simulink model "ABS_demo"  (R2022b)
settings: Solver=VariableStepAuto  StartTime=0.0  StopTime=25  RelTol=1e-3
undefined symbols (not defined in the file): g, I, m, R, v0
settings Model: Creator=Stephen Kingston  LastModifiedBy=OS
settings SolverCC: AlgebraicLoopSolver=TrustRegion
settings DebuggingCC: UnconnectedInputMsg=warning  UnconnectedOutputMsg=warning  UnconnectedLineMsg=warning  SFMachineParentedDataDiag=warning
settings ModelReferenceCC: EnableRefExpFcnMdlSchedulingChecks=on
settings SFSimCC: CustomCodeUndefinedFunction=UseInterfaceOnly

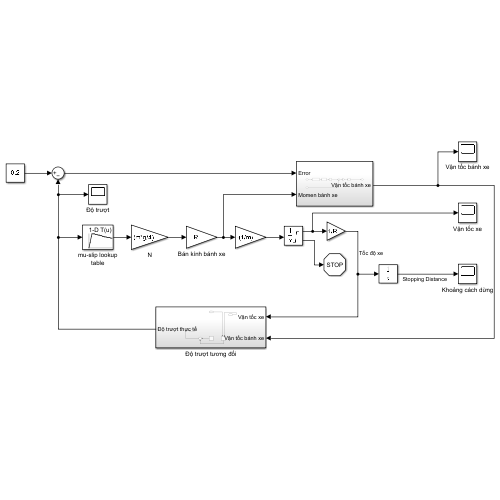
[thumbnail: Simulink's stored preview of the top-level diagram]
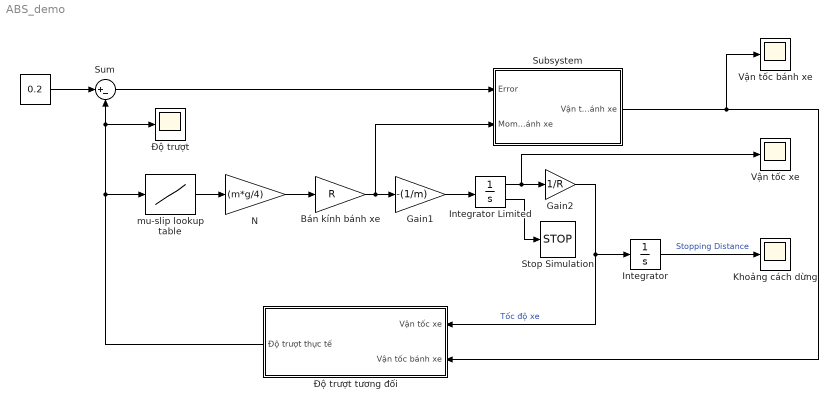
== system ABS_demo ==
  " " : Constant  Value=0.2
  Bán kính bánh xe : Gain  Gain=R
  Gain1 : Gain  Gain=-(1/m)
  Gain2 : Gain  Gain=1/R
  Integrator : Integrator
  Integrator Limited : Integrator  InitialCondition=v0  LimitOutput=on  UpperSaturationLimit=1000  LowerSaturationLimit=0  ShowSaturationPort=on
  Khoảng cách dừng : Scope
  N : Gain  Gain=(m*g/4)
  Stop Simulation : Stop
  Subsystem : Subsystem
  Sum : Sum  Inputs=|+-
  Vận tốc bánh xe : Scope
  Vận tốc xe : Scope
  mu-slip lookup table : Lookup_n-D  NumberOfTableDimensions=1  BreakpointsForDimension1=[0,0.05,0.1,0.15,0.2,0.25,0.3,0.35,0.4,0.45,0.5,0.55,0.60,0.65,0.70,0.75,0.80,0.85,0.90,0.95,1]  Table=[0,0.4,0.8,0.97,1,0.98,0.96,0.94,0.92,0.9,0.88,0.855,0.83,0.81,0.79,0.77,0.75,0.73,0.72,0.71,0.7]  InternalRulePriority=Speed  RndMeth=Simplest
  "Độ trượt " : Scope
  Độ trượt tương đối : Subsystem
  wires:
  Sum/1 -> Subsystem/1(Error)
  Bán kính bánh xe/1 -> Gain1/1, Subsystem/2(Momen bánh xe)
  Gain2/1 -> Độ trượt tương đối/1(Vận tốc xe), Integrator/1  "Tốc độ xe"
  " "/1 -> Sum/1
  mu-slip lookup table/1 -> N/1
  N/1 -> Bán kính bánh xe/1
  Gain1/1 -> Integrator Limited/1
  Integrator Limited/1 -> Vận tốc xe/1, Gain2/1
  Integrator/1 -> Khoảng cách dừng/1  "Stopping Distance"
  Integrator Limited/2 -> Stop Simulation/1
  Subsystem/1(Vận tốc bánh xe) -> Vận tốc bánh xe/1, Độ trượt tương đối/2(Vận tốc bánh xe)
  Độ trượt tương đối/1(Độ trượt thực tế) -> "Độ trượt "/1, Sum/2, mu-slip lookup table/1

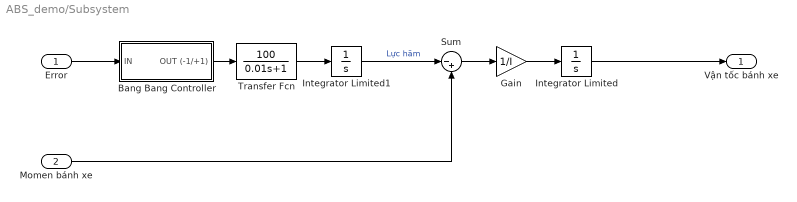
== system ABS_demo/Subsystem ==
  Error : Inport
  Momen bánh xe : Inport  Port=2
  Bang Bang Controller : Subsystem
  Gain : Gain  Gain=1/I
  Integrator Limited : Integrator  InitialCondition=v0/R  LimitOutput=on  UpperSaturationLimit=1000  LowerSaturationLimit=0
  Integrator Limited1 : Integrator  LimitOutput=on  UpperSaturationLimit=1500  LowerSaturationLimit=0
  Sum : Sum  Inputs=|-+
  Transfer Fcn : TransferFcn  Numerator=[100]  Denominator=[0.01 1]
  Vận tốc bánh xe : Outport  VectorParamsAs1DForOutWhenUnconnected=off
  wires:
  Sum/1 -> Gain/1
  Transfer Fcn/1 -> Integrator Limited1/1
  Gain/1 -> Integrator Limited/1
  Integrator Limited/1 -> Vận tốc bánh xe/1
  Integrator Limited1/1 -> Sum/1  "Lực hãm"
  Bang Bang Controller/1(OUT (-1/+1)) -> Transfer Fcn/1
  Momen bánh xe/1 -> Sum/2
  Error/1 -> Bang Bang Controller/1(IN)

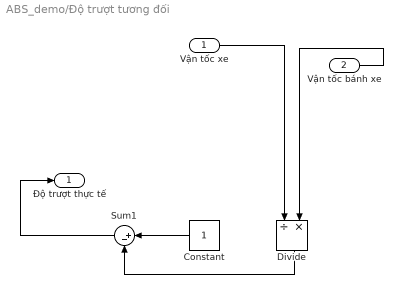
== system ABS_demo/Độ trượt tương đối ==
  Vận tốc xe : Inport
  Vận tốc bánh xe : Inport  Port=2
  Constant : Constant
  Divide : Product  Inputs=/*
  Sum1 : Sum  Inputs=|+-
  Độ trượt thực tế : Outport  VectorParamsAs1DForOutWhenUnconnected=off
  wires:
  Divide/1 -> Sum1/2
  Sum1/1 -> Độ trượt thực tế/1
  Constant/1 -> Sum1/1
  Vận tốc bánh xe/1 -> Divide/2
  Vận tốc xe/1 -> Divide/1

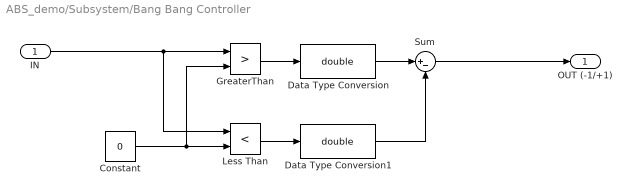
== system ABS_demo/Subsystem/Bang Bang Controller ==
  IN : Inport
  Constant : Constant  Value=0
  Data Type Conversion : DataTypeConversion  OutDataTypeStr=double  SaturateOnIntegerOverflow=off
  Data Type Conversion1 : DataTypeConversion  OutDataTypeStr=double  SaturateOnIntegerOverflow=off
  GreaterThan : RelationalOperator  Operator=>  OutDataTypeStr=boolean  RndMeth=Simplest  InputSameDT=off
  Less Than : RelationalOperator  Operator=<  OutDataTypeStr=boolean  RndMeth=Simplest  InputSameDT=off
  Sum : Sum  Inputs=|+-
  OUT (-1/+1) : Outport  VectorParamsAs1DForOutWhenUnconnected=off
  wires:
  Sum/1 -> OUT (-1/+1)/1
  Data Type Conversion/1 -> Sum/1
  Constant/1 -> GreaterThan/2, Less Than/2
  IN/1 -> Less Than/1, GreaterThan/1
  Data Type Conversion1/1 -> Sum/2
  GreaterThan/1 -> Data Type Conversion/1
  Less Than/1 -> Data Type Conversion1/1
